simulink model "WendVsMatern_MRAC"  (R2022b)
settings: Solver=ode45  StartTime=0.0  StopTime=30  RelTol=1e-3
values from neighbouring files (symbols this model uses):
  alpha0 = 0    [Run_Both_Model.m]    (also in Run_Deadzone.m; Run_ScalarModel.m; Slicing.m; UniCenterMRAC.m)
  ar = -20    [Run_Both_Model.m]    (also in Run_Deadzone.m; Run_Project1i_haoran9.m; Run_ScalarModel.m; Slicing.m)
  astar = -10    [Run_Both_Model.m]    (also in Run_Deadzone.m; Run_Project1i_haoran9.m; Run_ScalarModel.m; Slicing.m)
  beta0 = 0    [Run_Both_Model.m]    (also in Run_Deadzone.m; Run_ScalarModel.m; Slicing.m; UniCenterMRAC.m)
  br = 20    [Run_Both_Model.m]    (also in Run_Deadzone.m; Run_Project1i_haoran9.m; Run_ScalarModel.m; Slicing.m)
  bstar = +10    (= 10)    [Run_Both_Model.m]    (also in Run_Deadzone.m; Run_Project1i_haoran9.m; Run_ScalarModel.m; Slicing.m)
  centers = linspace(-OmegaLim-ext,OmegaLim+ext,N)'    [UniCenterMRAC.m]    (also in getOfflineError.m = linspace(-OmegaLim-ext,OmegaLim+ext,Ns(nn))'; getOfflineErrorNewt.m = linspace(-OmegaLim-ext,OmegaLim+ext,Ns(nn))'; getOfflineErrorNewt2.m = linspace(-OmegaLim-ext,OmegaLim+ext,Ns(nn))'; getVDP_HNorm.m = omegaCover2(Ri,Ro,h(hh)))
  ga = 10    [Run_Both_Model.m]    (also in Run_Deadzone.m; Run_ScalarModel.m; Slicing.m; UniCenterMRAC.m = 0)
  gb = 10    [Run_Both_Model.m]    (also in Run_Deadzone.m; Run_ScalarModel.m; Slicing.m; UniCenterMRAC.m = 0)
  gf = 10    [Run_Both_Model.m]    (also in Run_Deadzone.m; Run_ScalarModel.m; Slicing.m; UniCenterMRAC.m = 1)
  hyperMtrn = 2    [runMatern_MRAC.m]    (also in runWendVsMaternMRAC.m)
  hyperWend = 4    [runMatern_MRAC.m]    (also in runWendVsMaternMRAC.m = 5)
  invKMtrn = inv(KMtrn)    [runMatern_MRAC.m]    (also in runWendVsMaternMRAC.m)
  invKWend = inv(KWend)    [runWendVsMaternMRAC.m]
  nu = 1/2*(s+Dim/2)    (= 1)    [UniCenterMRAC.m]    (also in frbf.m = RBFpar; kernel2.m = par; runCompareBasisMRAC.m; runMatern_MRAC.m = 1.5)
  sig = 2    [Run_Both_Model.m]    (also in Run_Deadzone.m; Run_ScalarModel.m; Slicing.m; runMatern_MRAC.m)
  sigma = 0.1    [Run_Both_Model.m]    (also in Run_Deadzone.m; Run_Project1i_haoran9.m; Run_ScalarModel.m; Slicing.m)
  x0 = 0    [Run_Both_Model.m]    (also in Run_Deadzone.m; Run_Project1i_haoran9.m = 1; Run_ScalarModel.m; Slicing.m = 5)
  xr0 = 0    [Run_Both_Model.m]    (also in Run_Deadzone.m; Run_Project1i_haoran9.m; Run_ScalarModel.m; Slicing.m)
libraries: simulink x3
settings Model: Creator=owned  LastModifiedBy=Nathan
settings SolverCC: AlgebraicLoopSolver=TrustRegion
settings DebuggingCC: UnconnectedInputMsg=warning  UnconnectedOutputMsg=warning  UnconnectedLineMsg=warning  SFMachineParentedDataDiag=warning
settings ModelReferenceCC: EnableRefExpFcnMdlSchedulingChecks=on
settings RTWCC: DLArmComputeVersion=19.05

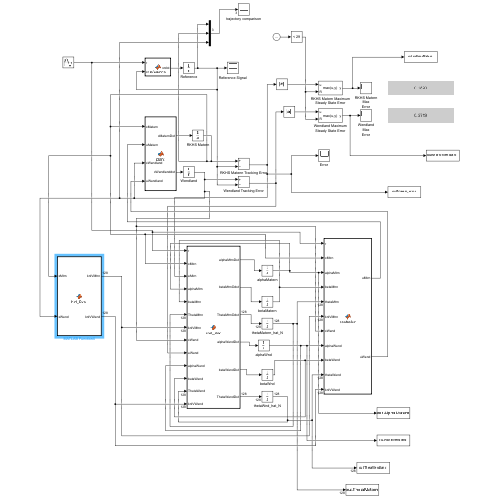
[thumbnail: Simulink's stored preview of the top-level diagram]
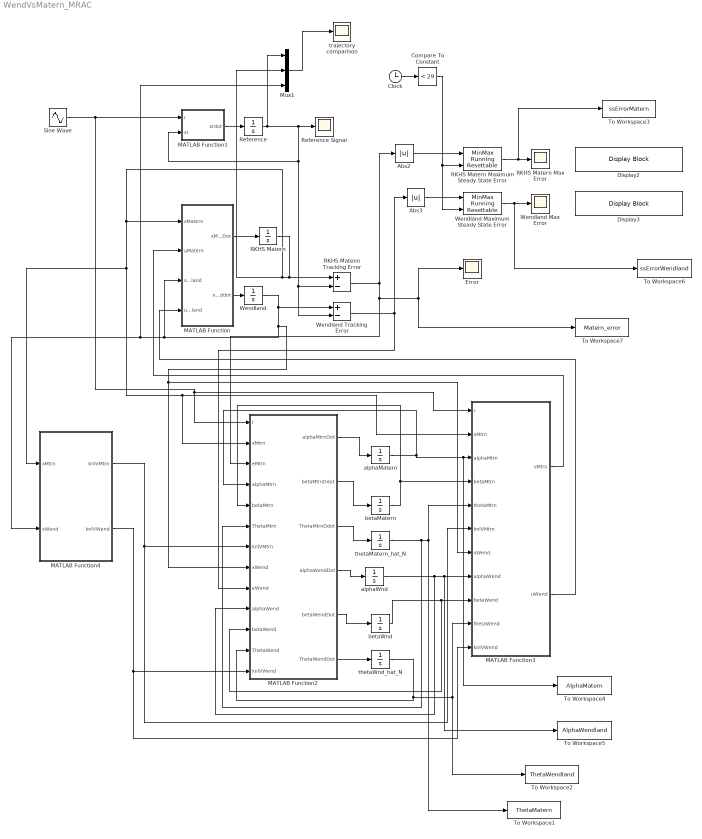
== system WendVsMatern_MRAC ==
  Abs2 : Abs  SaturateOnIntegerOverflow=off
  Abs3 : Abs  SaturateOnIntegerOverflow=off
  Clock : Clock
  Compare To Constant : simulink/Logic and Bit Operations/Compare To Constant  relop=<  const=29  OutDataTypeStr=boolean
  Display2 : DisplayBlock  LabelPosition=Hide  Transparency=1
  Display3 : DisplayBlock  LabelPosition=Hide  Transparency=1
  Error : Scope
  MATLAB Function : MATLAB Function  TreatAsAtomicUnit=on
  MATLAB Function1 : MATLAB Function  TreatAsAtomicUnit=on
  MATLAB Function2 : MATLAB Function  TreatAsAtomicUnit=on
  MATLAB Function3 : MATLAB Function  TreatAsAtomicUnit=on
  MATLAB Function4 : MATLAB Function  TreatAsAtomicUnit=on
  Mux1 : Mux  Inputs=3
  RKHS Matenn Tracking Error : Sum  Inputs=+-
  RKHS Matern : Integrator  InitialCondition=x0
  RKHS Matern Max Error : Scope
  RKHS Matern Maximum Steady State Error : simulink/Math Operations/MinMax Running Resettable  Function=max  vinit=0.0
  Reference : Integrator  InitialCondition=xr0
  Reference Signal : Scope
  Sine Wave : Sin  Amplitude=10  Frequency=2*pi  SampleTime=0
  To Workspace1 : ToWorkspace  VariableName=ThetaMatern  SaveFormat=Timeseries  SampleTime=-1
  To Workspace2 : ToWorkspace  VariableName=ThetaWendland  SaveFormat=Timeseries  SampleTime=-1
  To Workspace3 : ToWorkspace  VariableName=ssErrorMatern  SaveFormat=Timeseries  SampleTime=-1
  To Workspace4 : ToWorkspace  VariableName=AlphaMatern  SaveFormat=Timeseries  SampleTime=-1
  To Workspace5 : ToWorkspace  VariableName=AlphaWendland  SaveFormat=Timeseries  SampleTime=-1
  To Workspace6 : ToWorkspace  VariableName=ssErrorWendland  SaveFormat=Timeseries  SampleTime=-1
  To Workspace7 : ToWorkspace  VariableName=Matern_error  SaveFormat=Timeseries  SampleTime=-1
  Wendland : Integrator  InitialCondition=x0
  Wendland Max Error : Scope
  Wendland Maximum Steady State Error : simulink/Math Operations/MinMax Running Resettable  Function=max  vinit=0.0
  Wendland Tracking Error : Sum  Inputs=+-
  alphaMatern : Integrator  InitialCondition=alpha0
  alphaWnd : Integrator  InitialCondition=alpha0
  betaMatern : Integrator  InitialCondition=beta0
  betaWnd : Integrator  InitialCondition=beta0
  thetaMatern_hat_N : Integrator
  thetaWnd_hat_N : Integrator
  trajectory comparison : Scope
  wires:
  Sine Wave/1 -> MATLAB Function1/1(r), MATLAB Function2/1(r), MATLAB Function3/1(r)
  MATLAB Function1/1(xrdot) -> Reference/1
  Reference/1 -> Reference Signal/1, RKHS Matenn Tracking Error/2, Wendland Tracking Error/2, MATLAB Function1/2(xr), Mux1/1
  MATLAB Function/1(xMaternDot) -> RKHS Matern/1
  MATLAB Function/2(xWendlanddot) -> Wendland/1
  Wendland/1 -> MATLAB Function/3(xWendland), Mux1/3, MATLAB Function4/2(xWend), MATLAB Function2/8(xWend), MATLAB Function3/7(xWend), Wendland Tracking Error/1
  RKHS Matern/1 -> Mux1/2, MATLAB Function3/2(xMtrn), MATLAB Function2/2(xMtrn), MATLAB Function4/1(xMtrn), MATLAB Function/1(xMatern), RKHS Matenn Tracking Error/1
  RKHS Matenn Tracking Error/1 -> MATLAB Function2/3(eMtrn), To Workspace7/1, Error/1, Abs2/1
  Wendland Tracking Error/1 -> MATLAB Function2/9(eWend), Abs3/1
  MATLAB Function2/2(betaMtrnDdot) -> betaMatern/1
  MATLAB Function2/3(ThetaMtrnDdot) -> thetaMatern_hat_N/1
  MATLAB Function2/4(alphaWendDot) -> alphaWnd/1
  MATLAB Function2/5(betaWendDot) -> betaWnd/1
  MATLAB Function2/6(ThetaWendDot) -> thetaWnd_hat_N/1
  MATLAB Function4/2(knlVWend) -> MATLAB Function3/11(knlVWend), MATLAB Function2/13(knlVWend)
  alphaMatern/1 -> To Workspace4/1, MATLAB Function3/3(alphaMtrn), MATLAB Function2/4(alphaMtrn)
  betaMatern/1 -> MATLAB Function3/4(betaMtrn), MATLAB Function2/5(betaMtrn)
  thetaMatern_hat_N/1 -> MATLAB Function2/6(ThetaMtrn), To Workspace1/1, MATLAB Function3/5(thetaMtrn)
  alphaWnd/1 -> MATLAB Function2/10(alphaWend), To Workspace5/1, MATLAB Function3/8(alphaWend)
  betaWnd/1 -> MATLAB Function2/11(betaWend), MATLAB Function3/9(betaWend)
  thetaWnd_hat_N/1 -> To Workspace2/1, MATLAB Function3/10(thetaWend), MATLAB Function2/12(ThetaWend)
  MATLAB Function3/1(uMtrn) -> MATLAB Function/2(uMatern)
  MATLAB Function3/2(uWend) -> MATLAB Function/4(uWendland)
  Clock/1 -> Compare To Constant/1
  Compare To Constant/1 -> Wendland Maximum Steady State Error/2, RKHS Matern Maximum Steady State Error/2
  RKHS Matern Maximum Steady State Error/1 -> To Workspace3/1, RKHS Matern Max Error/1
  Wendland Maximum Steady State Error/1 -> To Workspace6/1, Wendland Max Error/1
  Abs2/1 -> RKHS Matern Maximum Steady State Error/1
  Abs3/1 -> Wendland Maximum Steady State Error/1
  Mux1/1 -> trajectory comparison/1
  MATLAB Function2/1(alphaMtrnDot) -> alphaMatern/1
  MATLAB Function4/1(knlVMtrn) -> MATLAB Function3/6(knlVMtrn), MATLAB Function2/7(knlVMtrn)

== matlab function WendVsMatern_MRAC/MATLAB Function3 ==
  data: r input; xMtrn input; alphaMtrn input; betaMtrn input; thetaMtrn input; knlVMtrn input; xWend input; alphaWend input; betaWend input; thetaWend input; knlVWend input; uMtrn output size=1; uWend output size=1
function [uMtrn, uWend]= controller(r, xMtrn,alphaMtrn,betaMtrn, thetaMtrn,knlVMtrn, xWend,alphaWend,betaWend, thetaWend,knlVWend)

% Matern 3/2
uMtrn = alphaMtrn*xMtrn+betaMtrn*r-thetaMtrn'*knlVMtrn;
% u3m = beta3m*r-theta3m'*knl_x3m;
% Matern 5/2
uWend = alphaWend*xWend+betaWend*r-thetaWend'*knlVWend;
% u5m = beta5m*r-theta5m'*knl_x5m;

== matlab function WendVsMatern_MRAC/MATLAB Function4 ==
  data: xMtrn input; xWend input; knlVMtrn output; centers parameter; hyperMtrn parameter; sig parameter; knlVWend output; nu parameter; hyperWend parameter
function [knlVMtrn,knlVWend] = Knl_Eval(xMtrn,xWend,centers,hyperMtrn,sig,nu, hyperWend)


% knlfun3m=@(x,bsc) sig^2.*(1+sqrt(3)./hyper.*abs(x-bsc)).*exp(-sqrt(3).*abs(x-bsc)./hyper);
% knlfun5m=@(x,bsc) sig^2.*(1+sqrt(5)/hyperMatern.*abs(x-bsc)+5/(3*hyperMatern^2).*abs(x-bsc).^2).*exp(-sqrt(5).*abs(x-bsc)./hyperMatern);

knlfuncMtrn=@(r) real(sig^2*2^(1-nu)/gamma(nu)*(sqrt(2*nu)*r/hyperMtrn)^nu*besselk(nu,sqrt(2*nu)*r/hyperMtrn));
knlfuncWend=@(r) (1-r/hyperWend)^6*(35*(r/hyperWend)^2 + 18*r/hyperWend +3);


knlVMtrn=zeros(length(centers),1);
knlVWend=zeros(length(centers),1);

for ii=1:length(centers)
    rM = abs(xMtrn-centers(ii));
    if rM > 1e-12
        knlVMtrn(ii)=knlfuncMtrn(rM);
    else 
        knlVMtrn(ii)= 1;
    end   
    rW = abs(xWend-centers(ii));
    if 1-rW/hyperWend <= 0
        knlVWend(ii) = 0;
    else 
        knlVWend(ii)= knlfuncWend(rW);
    end 
end

== matlab function WendVsMatern_MRAC/MATLAB Function1 ==
  data: r input; xr input; xrdot output; ar parameter; br parameter
function xrdot = reference(r,xr,ar, br)

xrdot = ar*xr+br*r;

== matlab function WendVsMatern_MRAC/MATLAB Function ==
  data: xMatern input; uMatern input; xWendland input; uWendland input; astar parameter; bstar parameter; xMaternDot output; xWendlanddot output
function [xMaternDot,xWendlanddot] = plant(xMatern,uMatern,xWendland,uWendland,astar, bstar)


xMaternDot = astar*xMatern+bstar*(uMatern+10*tanh(xMatern));
xWendlanddot = astar*xWendland+bstar*(uWendland+10*tanh(xWendland));

== matlab function WendVsMatern_MRAC/MATLAB Function2 ==
  data: ga parameter; gb parameter; gf parameter; sigma parameter; alphaMtrnDot output size=1; betaMtrnDdot output size=1; ThetaMtrnDdot output size=N; alphaWendDot output size=1; betaWendDot output size=1; ThetaWendDot output size=N; r input; xMtrn input; eMtrn input; alphaMtrn input; betaMtrn input; ThetaMtrn input; knlVMtrn input; xWend input; eWend input; alphaWend input; betaWend input; ThetaWend input; knlVWend input; invKMtrn parameter; invKWend parameter
function [alphaMtrnDot, betaMtrnDdot, ThetaMtrnDdot, alphaWendDot, betaWendDot, ThetaWendDot] = evo_law(ga, gb, gf, sigma, r, xMtrn, eMtrn, alphaMtrn, betaMtrn, ThetaMtrn, knlVMtrn, xWend, eWend, alphaWend, betaWend, ThetaWend, knlVWend, invKMtrn, invKWend)

%% Matern Standard RKHS
alphaMtrnDot=-ga*xMtrn*eMtrn-sigma*alphaMtrn;
betaMtrnDdot=-gb*r*eMtrn-sigma*betaMtrn;
ThetaMtrnDdot=gf*invKMtrn*knlVMtrn*eMtrn-sigma*ThetaMtrn;
%% Wendland 32 Standard RKHS
alphaWendDot=-ga*xWend*eWend-sigma*alphaWend;
betaWendDot=-gb*r*eWend-sigma*betaWend;
ThetaWendDot=gf*invKWend*knlVWend*eWend-sigma*ThetaWend;
